simulink model "exam_model_R2020a_final"  (R2022a)
settings: Solver=VariableStepAuto  StartTime=0.0  StopTime=120  FixedStep=inc  MaxStep=1e-2  EnableMultiTasking=on
undefined symbols (not defined in the file): B, C, converter_const, J, ki, kiw, kp, kpw, kpw_load, L, L_f, R_f, R_L, T_load, Vin
settings Model: Creator=Dave  LastModifiedBy=aasav
settings SolverCC: AlgebraicLoopSolver=TrustRegion
settings DataIOCC: LimitDataPoints=on  SaveFormat=Array  SignalLoggingSaveFormat=ModelDataLogs  LoggingToFile=on
settings OptimizationCC: ExpressionDepthLimit=2147483647  InitFltsAndDblsToZero=on  LifeSpan=inf
settings DebuggingCC: SaveWithParameterizedLinksMsg=none  UnderspecifiedInitializationDetection=Classic  MergeDetectMultiDrivingBlocksExec=none  SolverPrmCheckMsg=warning  FcnCallInpInsideContextMsg=warning  UnconnectedInputMsg=warning  UnconnectedOutputMsg=warning  UnconnectedLineMsg=warning  StateNameClashWarn=warning  SFUnexpectedBacktrackingDiag=warning  SFNoUnconditionalDefaultTransitionDiag=warning  SFExecutionAtInitializationDiag=none  SFMachineParentedDataDiag=warning  ArithmeticOperatorsInVariantConditions=warning
settings HardwareCC: ProdBitPerPointer=32  ProdBitPerSizeT=32  ProdBitPerPtrDiffT=32  ProdLargestAtomicFloat=None  ProdIntDivRoundTo=Undefined  ProdEndianess=Unspecified  ProdWordSize=32  ProdHWDeviceType=32-bit Generic
settings ModelReferenceCC: PropagateSignalLabelsOutOfModel=off
settings CodeAppCC: StateflowObjectComments=on
settings GRTTargetCC: TargetLangStandard=C89/C90 (ANSI)  CombineOutputUpdateFcns=off  GRTInterface=on
settings ConfigComp: CovMetricSettings=dw  CovSaveCumulativeToWorkspaceVar=on  CovSaveSingleToWorkspaceVar=on

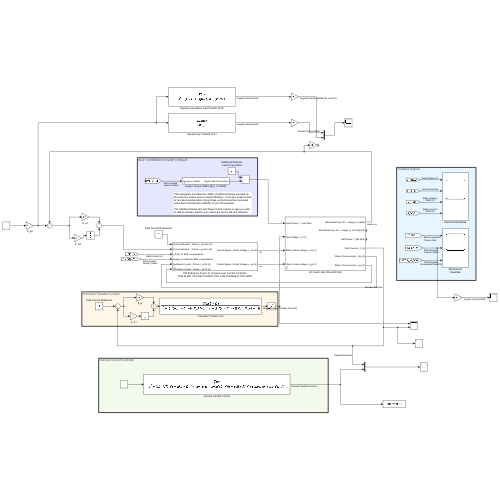
[thumbnail: Simulink's stored preview of the top-level diagram]
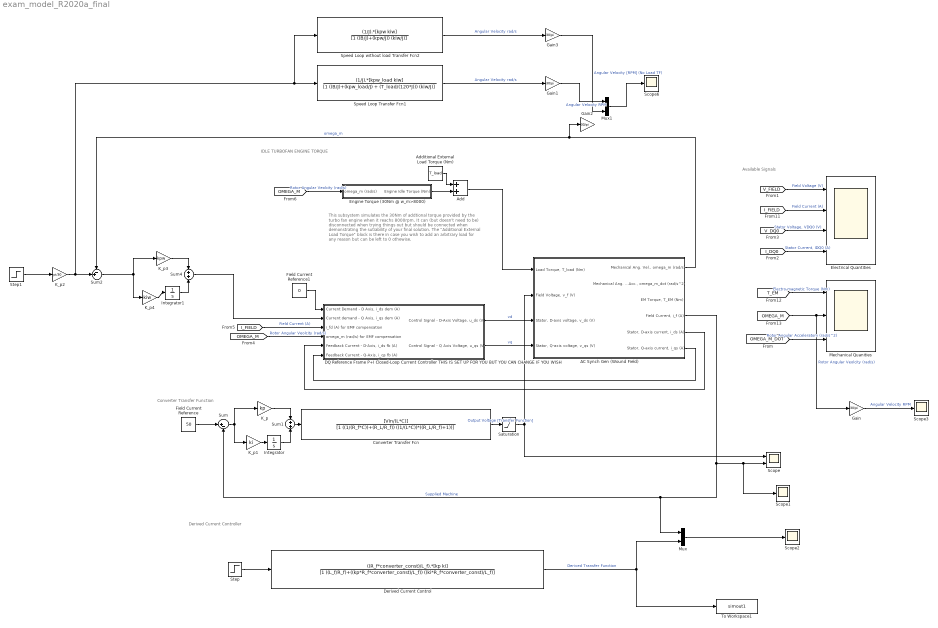
== system exam_model_R2020a_final ==
  note: Converter Transfer Function
  note: Derived Current Controller
  note: This subsystem simulates the 30Nm of addtional torque provided by the turbo fan engine when it reachs 8000rpm.  It can (but doesn't need to be) disconnected when trying things out but should be connected when demonstrating the sutiability of your final solution.
      |
      | The "Additional External Load Torque" block is there in case you wish to add an arbitrary load for any reason but can be left to 0 othewise.
  note: IDLE TURBOFAN ENGINE TORQUE
  note: Available Signals
  AC Synch Gen (Wound Field) : Subsystem  mask(Synchronous Generator Model (No Saturation)){J_rotor=0.5, B_viscous=0.05, Pole_Pairs=3, Ns_by_Nf=0.3, wind_const=1.5, R_s=0.04, L_s=5e-5, L_d=0.00057, R_fd_p=0.223*1.5*0.3^2, L_fd_p=0.0138*1.5*0.3^2, L_q=0.00032}
      mask prompts: J_rotor "Rotor Mass Moment-of-Interia, J_rotor, kg m^2"; B_viscous "Rotor Viscous Friction Coefficient, B_viscous (Nm s/rad)"; Pole_Pairs "Rotor Pole Pairs"; Ns_by_Nf "Stator to Field Turns Ratio, Ns_by_Nf"; wind_const "Winding Constant (Normally 1.5)"; R_s "Stator Resistance, R_s (Ohms)"; L_s "Stator Leakage Inductance, L_s (H)"; L_d "D-Axis Synchronous Inductance, L_d (H)"; R_fd_p "Referred Field Resistance, R_fd_p (Ohms)"; L_fd_p "Referred Field Leakage Inducatnce, L_fd_p (H)"; L_q "Q-Axis Synchronous Inductance, L_q (H)"
      mask help: Standard SI units version of a Would Field Synchronous Generator. All rotor parameters must be supplied referred from the rotor side to the stator.
      mask init:
      | L_md = L_d - L_s
      | L_MD_TOTAL = 1 / ( ( 1/L_md ) + ( 1/L_fd_p ) + ( 1/L_s ) )
      | L_mq = L_q - L_s
      | L_MQ_TOTAL = 1 / ( ( 1/L_mq ) + ( 1/L_s ) )
      mask DialogControl Container4 Prompt: Mechanical Parameters
      mask DialogControl Container6 Prompt: Electrical Parameters
      mask DialogControl Container8 Prompt: General
      mask DialogControl Container13 Prompt: Stator Synchronous Parameters
      mask DialogControl Container9 Prompt: D-Axis Parameters
      mask DialogControl Container11 Prompt: Referred Field Winding
      mask DialogControl Container10 Prompt: Q-Axis Parameters
  Add : Sum
  Additional External Load Torque (Nm) : Constant  Value=T_load
  Converter Transfer Fcn : TransferFcn  Numerator=[Vin/(L*C)]  Denominator=[1 ((1/(R_f*C))+(R_L/R_f)) ((1/(L*C))*((R_L/R_f)+1))]
  DQ Reference Frame P+I Closed-Loop Current Controller THIS IS SET UP FOR YOU BUT YOU CAN CHANGE IF YOU WISH : Subsystem  mask{emfcomp=on, kp_d=5, ki_d=20, kp_q=3, ki_q=15}
      mask prompts: emfcomp "Current Controller EMF Compensation?"; kp_d "d-Axis Proportional Gain"; ki_d "d-Axis Integral Gain"; kp_q "q-Axis Proportional Gain"; ki_q "q-axis Integral Gain"
      mask help:
      | A simple two axis feedback controller based upon a P + I structure.
      |
      | NOTE: The block simply implements two independent P + I controllers with no saturation or integrator anti-wind up protection.  Controller Gains are set in this dialog box.
      |
      | There is the option of using EMF Compesnation to simplfy controller design.  When enabled the EMF is added to the relevant axis of the machine winding to ensure that the controller is only providivng a voltage over and above this value, this simplifies controller design over a wide speed range.
      mask DialogControl Container5 Prompt: Current Controller
      mask DialogControl ParameterGroupVar Prompt: Current Controller Gains
      mask DialogControl Container4 Prompt: D-Axis P+I Controller Gains
      mask DialogControl Container3 Prompt: Q-Axis P+I Controller Gains
  Derived Current Control : TransferFcn  Numerator=((R_f*converter_const)/L_f).*[kp ki]  Denominator=[1 ((L_f/R_f)+((kp*R_f*converter_const)/L_f)) ((ki*R_f*converter_const)/L_f)]
  Electrical Quantities : Scope  NumInputPorts=4
  Engine Torque (30Nm @ w_m>8000) : Subsystem  mask(Engine Idle Torque Simulation (Once lit)){idle_speed=8000, idle_torque=30}
      mask prompts: idle_speed "Engine Ignition Speed (rev/min)"; idle_torque "Engine Idle Torque (Nm)"
      mask help:
      | This subsystem simulates the 30Nm of addtional torque provided by the turbo fan engine when the engine shaft reaches  8000rpm and the engine ignites.  It can (but doesn't need to be) disconnected when trying things out but should be connected when demonstrating the sutiability of your final solution.
      |
      | The "Additional External Load Torque" block is there in case you wish to add an arbitrary load for any reason but can be left to 0 othewise.
  Field Current Reference : Constant  Value=50
  Field Current Reference1 : Constant  Value=0
  Gain{,1..3} (4 alike) : Gain  Gain=30/pi
  Integrator : Integrator
  Integrator1 : Integrator
  K_p : Gain  Gain=kp
  K_p1 : Gain  Gain=ki
  K_p2 : Gain  Gain=pi/30
  K_p3 : Gain  Gain=kpw
  K_p4 : Gain  Gain=kiw
  Mechanical Quanities : Scope  NumInputPorts=3
  Mux : Mux  Inputs=2
  Mux1 : Mux  Inputs=2
  Saturation : Saturate  UpperLimit=Vin*0.9  LowerLimit=0
  Scope : Scope  NumInputPorts=2
  Scope{1..3,6} (4 alike) : Scope
  Speed Loop Transfer Fcn1 : TransferFcn  Numerator=(1/J).*[kpw_load kiw]  Denominator=[1 ((B/J)+(kpw_load/J) + (T_load/(120*J))) (kiw/J)]
  Speed Loop without load Transfer Fcn2 : TransferFcn  Numerator=(1/J).*[kpw kiw]  Denominator=[1 ((B/J)+(kpw/J)) (kiw/J)]
  Step : Step  Time=0  After=50  SampleTime=0
  Step1 : Step  Time=5  After=12000  SampleTime=0
  Sum : Sum  Inputs=|+-
  Sum1 : Sum  Inputs=+|+
  Sum2 : Sum  Inputs=-+|
  Sum4 : Sum  Inputs=+|+
  To Workspace1 : ToWorkspace  VariableName=simout1  SaveFormat=Timeseries  SampleTime=-1
  wires:
  [OMEGA_M_DOT] -> Mechanical Quanities/3  "Rotor Angular Acceleratom (rad/s^2)"
  [I_DQ0] -> Electrical Quantities/4  "Stator Current, IDQ0 (A)"
  [V_DQ0] -> Electrical Quantities/3  "Stator Voltage, VDQ0 (V)"
  [I_FIELD] -> Electrical Quantities/2  "Field Current (A)"
  [V_FIELD] -> Electrical Quantities/1  "Field Voltage (V)"
  [T_EM] -> Mechanical Quanities/1  "Electro-magnetic Torque (Nm)"
  [OMEGA_M] -> Gain/1, Mechanical Quanities/2  "Rotor Angular Veolcity (rad/s)"
  AC Synch Gen (Wound Field)/6("Stator, Q-axis current, i_qs (A)") -> DQ Reference Frame P+I Closed-Loop Current Controller THIS IS SET UP FOR YOU BUT YOU CAN CHANGE IF YOU WISH/6("Feedback Current - Q-Axis, i_qs fb (A)")
  AC Synch Gen (Wound Field)/5("Stator, D-axis current, i_ds (A)") -> DQ Reference Frame P+I Closed-Loop Current Controller THIS IS SET UP FOR YOU BUT YOU CAN CHANGE IF YOU WISH/5("Feedback Current - D-Axis, i_ds fb (A)")
  DQ Reference Frame P+I Closed-Loop Current Controller THIS IS SET UP FOR YOU BUT YOU CAN CHANGE IF YOU WISH/1("Control Signal - D-Axis Voltage, u_ds (V)") -> AC Synch Gen (Wound Field)/3("Stator, D-axis voltage, v_ds (V)")  "vd"
  DQ Reference Frame P+I Closed-Loop Current Controller THIS IS SET UP FOR YOU BUT YOU CAN CHANGE IF YOU WISH/2("Control Signal - Q Axis Voltage, u_qs (V)") -> AC Synch Gen (Wound Field)/4("Stator, Q-axis voltage, v_qs (V)")  "vq"
  Add/1 -> AC Synch Gen (Wound Field)/1("Load Torque, T_load (Nm)")
  Additional External Load Torque (Nm)/1 -> Add/1
  Engine Torque (30Nm @ w_m>8000)/1(Engine Idle Torque (Nm)) -> Add/2
  [OMEGA_M] -> DQ Reference Frame P+I Closed-Loop Current Controller THIS IS SET UP FOR YOU BUT YOU CAN CHANGE IF YOU WISH/4(omega_m (rad/s) for EMF compensation)  "Rotor Angular Veolcity (rad/s)"
  [I_FIELD] -> DQ Reference Frame P+I Closed-Loop Current Controller THIS IS SET UP FOR YOU BUT YOU CAN CHANGE IF YOU WISH/3(i_fd (A) for EMF compensation)  "Field Current (A)"
  [OMEGA_M] -> Engine Torque (30Nm @ w_m>8000)/1(omega_m (rad/s))  "Rotor Angular Veolcity (rad/s)"
  Converter Transfer Fcn/1 -> Saturation/1  "Output Voltage [Transfer Function]"
  AC Synch Gen (Wound Field)/4("Field Current, i_f (A)") -> Mux/1, Sum/2, Scope1/1, Scope/2  "Supplied Machine"
  Field Current Reference/1 -> Sum/1
  K_p/1 -> Sum1/1
  Sum1/1 -> Converter Transfer Fcn/1
  Saturation/1 -> AC Synch Gen (Wound Field)/2("Field Voltage, v_f (V)"), Scope/1
  Sum/1 -> K_p1/1, K_p/1
  Integrator/1 -> Sum1/2
  K_p1/1 -> Integrator/1
  Step/1 -> Derived Current Control/1
  Derived Current Control/1 -> Mux/2, To Workspace1/1  "Derived Transfer Function"
  Mux/1 -> Scope2/1
  K_p2/1 -> Speed Loop without load Transfer Fcn2/1, Speed Loop Transfer Fcn1/1, Sum2/2
  Step1/1 -> K_p2/1
  AC Synch Gen (Wound Field)/1("Mechanical Ang. Vel., omega_m (rad/s)") -> Gain2/1, Sum2/1  "omega_m"
  K_p3/1 -> Sum4/1
  Sum2/1 -> K_p4/1, K_p3/1
  Integrator1/1 -> Sum4/2
  K_p4/1 -> Integrator1/1
  Sum4/1 -> DQ Reference Frame P+I Closed-Loop Current Controller THIS IS SET UP FOR YOU BUT YOU CAN CHANGE IF YOU WISH/2("Current demand - Q Axis, i_qs dem (A)")
  Field Current Reference1/1 -> DQ Reference Frame P+I Closed-Loop Current Controller THIS IS SET UP FOR YOU BUT YOU CAN CHANGE IF YOU WISH/1("Current Demand - D Axis, i_ds dem (A)")
  Gain/1 -> Scope3/1  "Angular Velocity RPM"
  Speed Loop Transfer Fcn1/1 -> Gain1/1  "Angular Velocity rad/s"
  Gain1/1 -> Mux1/1  "Angular Velocity RPM"
  Mux1/1 -> Scope6/1
  Speed Loop without load Transfer Fcn2/1 -> Gain3/1  "Angular Velocity rad/s"
  Gain3/1 -> Mux1/2  "Angular Velocity [RPM] (No Load TF)"

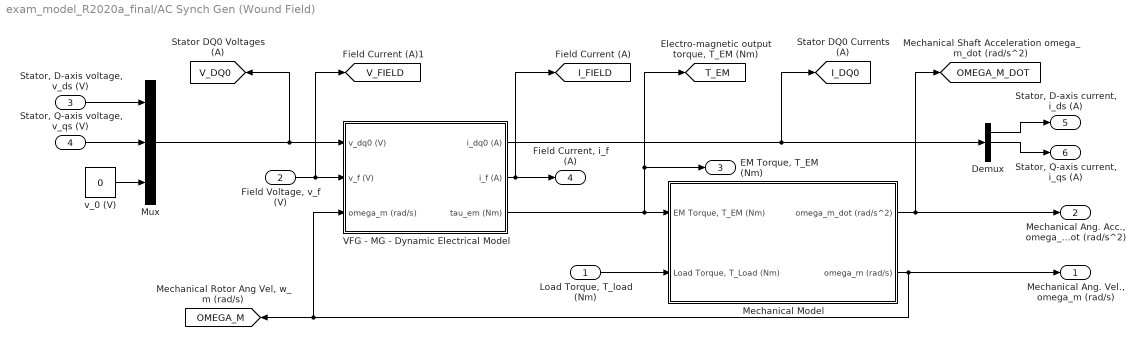
== system exam_model_R2020a_final/AC Synch Gen (Wound Field) ==
  "Load Torque, T_load (Nm)" : Inport
  "Field Voltage, v_f (V)" : Inport  Port=2
  "Stator, D-axis voltage, v_ds (V)" : Inport  Port=3
  "Stator, Q-axis voltage, v_qs (V)" : Inport  Port=4
  Demux : Demux  Outputs=3
  Mechanical Model : Subsystem  mask{Pole_Pairs=Pole_Pairs, J_rotor=J_rotor, B_viscous=B_viscous}
      mask prompts: Pole_Pairs "Rotor Pole Pairs"; J_rotor "Rotor Mass Moment-of-Inertia, J (kg m^2)"; B_viscous "Rotor Viscous Friction Constant, B_viscous (Nm s/rad)"
      mask DialogControl Container3 Prompt: Synchronous Generator Rotor Mechanical Parameters
  Mux : Mux  Inputs=3
  VFG - MG - Dynamic Electrical Model : Subsystem  mask{Pole_Pairs=Pole_Pairs, wind_const=wind_const, Ns_by_Nf=Ns_by_Nf, R_s=R_s, L_s=L_s, L_d=L_d, R_fd_p=R_fd_p, L_fd_p=L_fd_p, L_q=L_q}
      mask prompts: Pole_Pairs "Pole Pairs"; wind_const "Winding Constant"; Ns_by_Nf "Stator to Field Turns Ratio (Ns/Nf)"; R_s "Stator Resistance, R_s (Ohms)"; L_s "Stator Inductance, L_s (H)"; L_d "D-Axis Synchronous Inductance, L_d (H)"; R_fd_p "Referred Field Resistance, R_f_p (Ohms)"; L_fd_p "Referred Field Inductance, L_fd_p (H)"; L_q "Q-Axis Sychronous Inductance, L_q (H)"
      mask DialogControl Container4 Prompt: General Parameters
      mask DialogControl Container5 Prompt: D-Axis Parameters
      mask DialogControl Container8 Prompt: Referred Field
      mask DialogControl Container6 Prompt: Q-Axis Parameters
  v_0 (V) : Constant  Value=0
  "Mechanical Ang. Vel., omega_m (rad/s)" : Outport
  "Mechanical Ang. Acc., omega_m_dot (rad/s^2)" : Outport  Port=2
  "EM Torque, T_EM (Nm)" : Outport  Port=3
  "Field Current, i_f (A)" : Outport  Port=4
  "Stator, D-axis current, i_ds (A)" : Outport  Port=5
  "Stator, Q-axis current, i_qs (A)" : Outport  Port=6
  tag scope: I_DQ0=global, I_FIELD=global, OMEGA_M=global, OMEGA_M_DOT=global, T_EM=global, V_DQ0=global, V_FIELD=global
  wires:
  VFG - MG - Dynamic Electrical Model/1(i_dq0 (A)) -> Demux/1, [I_DQ0]
  "Field Voltage, v_f (V)"/1 -> [V_FIELD], VFG - MG - Dynamic Electrical Model/2(v_f (V))
  Mechanical Model/2(omega_m (rad/s)) -> [OMEGA_M], VFG - MG - Dynamic Electrical Model/3(omega_m (rad/s)), "Mechanical Ang. Vel., omega_m (rad/s)"/1
  VFG - MG - Dynamic Electrical Model/2(i_f (A)) -> [I_FIELD], "Field Current, i_f (A)"/1
  VFG - MG - Dynamic Electrical Model/3(tau_em (Nm)) -> [T_EM], "EM Torque, T_EM (Nm)"/1, Mechanical Model/1("EM Torque, T_EM (Nm)")
  "Load Torque, T_load (Nm)"/1 -> Mechanical Model/2("Load Torque, T_Load (Nm)")
  "Stator, D-axis voltage, v_ds (V)"/1 -> Mux/1
  "Stator, Q-axis voltage, v_qs (V)"/1 -> Mux/2
  v_0 (V)/1 -> Mux/3
  Mux/1 -> [V_DQ0], VFG - MG - Dynamic Electrical Model/1(v_dq0 (V))
  Demux/1 -> "Stator, D-axis current, i_ds (A)"/1
  Demux/2 -> "Stator, Q-axis current, i_qs (A)"/1
  Mechanical Model/1(omega_m_dot (rad/s^2)) -> [OMEGA_M_DOT], "Mechanical Ang. Acc., omega_m_dot (rad/s^2)"/1

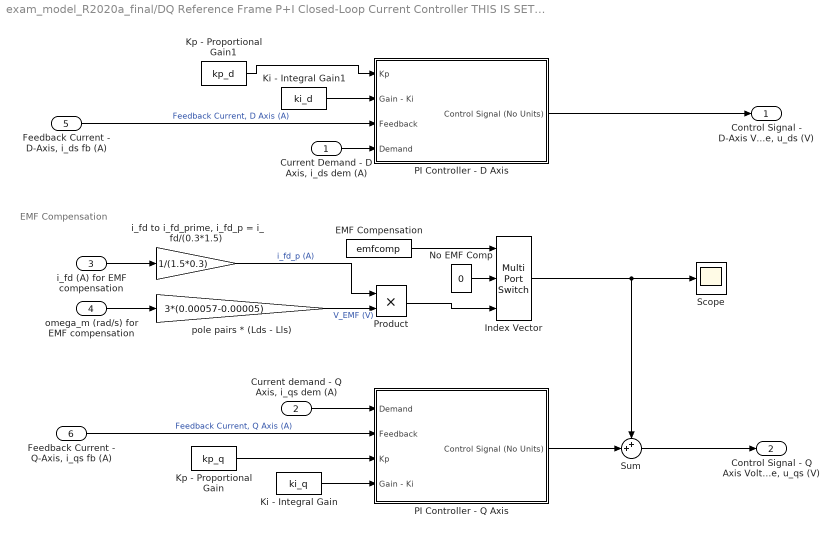
== system exam_model_R2020a_final/DQ Reference Frame P+I Closed-Loop Current Controller THIS IS SET UP FOR YOU BUT YOU CAN CHANGE IF YOU WISH ==
  note: EMF Compensation
  "Current Demand - D Axis, i_ds dem (A)" : Inport
  "Current demand - Q Axis, i_qs dem (A)" : Inport  Port=2
  i_fd (A) for EMF compensation : Inport  Port=3
  omega_m (rad/s) for EMF compensation : Inport  Port=4
  "Feedback Current - D-Axis, i_ds fb (A)" : Inport  Port=5
  "Feedback Current - Q-Axis, i_qs fb (A)" : Inport  Port=6
  EMF Compensation : Constant  Value=emfcomp
  Index Vector : MultiPortSwitch  DataPortOrder=Zero-based contiguous  Inputs=2  zeroidx=on  SaturateOnIntegerOverflow=off  InputSameDT=off
  Ki - Integral Gain : Constant  Value=ki_q
  Ki - Integral Gain1 : Constant  Value=ki_d
  Kp - Proportional Gain : Constant  Value=kp_q
  Kp - Proportional Gain1 : Constant  Value=kp_d
  No EMF Comp : Constant  Value=0
  PI Controller - D Axis : Subsystem  TreatAsAtomicUnit=on
  PI Controller - Q Axis : Subsystem  TreatAsAtomicUnit=on
  Product : Product
  Scope : Scope
  Sum : Sum  Inputs=++|
  "i_fd to i_fd_prime, i_fd_p = i_fd/(0.3*1.5)" : Gain  Gain=1/(1.5*0.3)
  pole pairs * (Lds - Lls) : Gain  Gain=3*(0.00057-0.00005)
  "Control Signal - D-Axis Voltage, u_ds (V)" : Outport  VectorParamsAs1DForOutWhenUnconnected=off
  "Control Signal - Q Axis Voltage, u_qs (V)" : Outport  Port=2  VectorParamsAs1DForOutWhenUnconnected=off
  wires:
  "Current demand - Q Axis, i_qs dem (A)"/1 -> PI Controller - Q Axis/1(Demand)
  "Feedback Current - Q-Axis, i_qs fb (A)"/1 -> PI Controller - Q Axis/2(Feedback)  "Feedback Current, Q Axis (A)"
  "Feedback Current - D-Axis, i_ds fb (A)"/1 -> PI Controller - D Axis/3(Feedback)  "Feedback Current, D Axis (A)"
  "Current Demand - D Axis, i_ds dem (A)"/1 -> PI Controller - D Axis/4(Demand)
  PI Controller - Q Axis/1(Control Signal (No Units)) -> Sum/2
  pole pairs * (Lds - Lls)/1 -> Product/2  "V_EMF (V)"
  Sum/1 -> "Control Signal - Q Axis Voltage, u_qs (V)"/1
  omega_m (rad/s) for EMF compensation/1 -> pole pairs * (Lds - Lls)/1
  EMF Compensation/1 -> Index Vector/1
  No EMF Comp/1 -> Index Vector/2
  Index Vector/1 -> Sum/1, Scope/1
  PI Controller - D Axis/1(Control Signal (No Units)) -> "Control Signal - D-Axis Voltage, u_ds (V)"/1
  Kp - Proportional Gain/1 -> PI Controller - Q Axis/3(Kp)
  Ki - Integral Gain/1 -> PI Controller - Q Axis/4(Gain - Ki)
  Kp - Proportional Gain1/1 -> PI Controller - D Axis/1(Kp)
  Ki - Integral Gain1/1 -> PI Controller - D Axis/2(Gain - Ki)
  i_fd (A) for EMF compensation/1 -> "i_fd to i_fd_prime, i_fd_p = i_fd/(0.3*1.5)"/1
  "i_fd to i_fd_prime, i_fd_p = i_fd/(0.3*1.5)"/1 -> Product/1  "i_fd_p (A)"
  Product/1 -> Index Vector/3

== system exam_model_R2020a_final/Engine Torque (30Nm @ w_m>8000) ==
  omega_m (rad/s) : Inport
  Engine Idle Torque Magnitude (Nm) : Constant  Value=idle_torque
  Engine Ignition Speed (rev/min) : Constant  Value=idle_speed
  Gain : Gain  Gain=2*pi/60
  Gain1 : Gain  Gain=-1
  Product : Product
  Relational Operator : RelationalOperator  OutDataTypeStr=boolean  RndMeth=Simplest  InputSameDT=off
  Engine Idle Torque (Nm) : Outport
  wires:
  Gain/1 -> Relational Operator/2
  Engine Idle Torque Magnitude (Nm)/1 -> Gain1/1
  Product/1 -> Engine Idle Torque (Nm)/1
  Relational Operator/1 -> Product/2
  omega_m (rad/s)/1 -> Relational Operator/1
  Engine Ignition Speed (rev/min)/1 -> Gain/1
  Gain1/1 -> Product/1

== system exam_model_R2020a_final/AC Synch Gen (Wound Field)/Mechanical Model ==
  note: T_Net = T_EM - T_Load
      | T_Net = (J * omega_m_dot) + (B * omega_m)
  "EM Torque, T_EM (Nm)" : Inport
  "Load Torque, T_Load (Nm)" : Inport  Port=2
  Gain : Gain  Gain=1/J_rotor
  Gain1 : Gain  Gain=B_viscous
  Integrator : Integrator
  Sum : Sum  Inputs=+--
  omega_m_dot (rad/s^2) : Outport
  omega_m (rad/s) : Outport  Port=2
  wires:
  "Load Torque, T_Load (Nm)"/1 -> Sum/2
  Sum/1 -> Gain/1  "Net Torque, T_net (Nm)"
  "EM Torque, T_EM (Nm)"/1 -> Sum/1
  Integrator/1 -> Gain1/1, omega_m (rad/s)/1  "omega_m (rad/s)"
  Gain/1 -> omega_m_dot (rad/s^2)/1, Integrator/1  "omega_m_dot (rad/s)"
  Gain1/1 -> Sum/3  "Viscous Friction Torque, T_fric (Nm)"

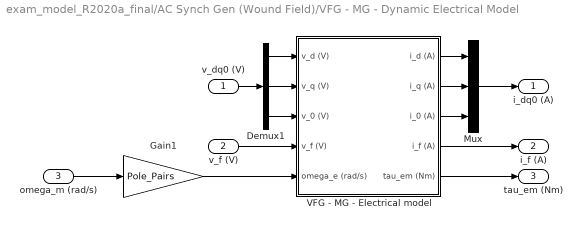
== system exam_model_R2020a_final/AC Synch Gen (Wound Field)/VFG - MG - Dynamic Electrical Model ==
  v_dq0 (V) : Inport
  v_f (V) : Inport  Port=2
  omega_m (rad/s) : Inport  Port=3
  Demux1 : Demux  Outputs=3
  Gain1 : Gain  Gain=Pole_Pairs
  Mux : Mux  Inputs=3
  VFG - MG - Electrical model : Subsystem
  i_dq0 (A) : Outport
  i_f (A) : Outport  Port=2
  tau_em (Nm) : Outport  Port=3
  wires:
  VFG - MG - Electrical model/4(i_f (A)) -> i_f (A)/1
  VFG - MG - Electrical model/5(tau_em (Nm)) -> tau_em (Nm)/1
  v_dq0 (V)/1 -> Demux1/1
  Mux/1 -> i_dq0 (A)/1
  omega_m (rad/s)/1 -> Gain1/1
  Gain1/1 -> VFG - MG - Electrical model/5(omega_e (rad/s))
  Demux1/1 -> VFG - MG - Electrical model/1(v_d (V))
  Demux1/2 -> VFG - MG - Electrical model/2(v_q (V))
  Demux1/3 -> VFG - MG - Electrical model/3(v_0 (V))
  v_f (V)/1 -> VFG - MG - Electrical model/4(v_f (V))
  VFG - MG - Electrical model/1(i_d (A)) -> Mux/1
  VFG - MG - Electrical model/2(i_q (A)) -> Mux/2
  VFG - MG - Electrical model/3(i_0 (A)) -> Mux/3

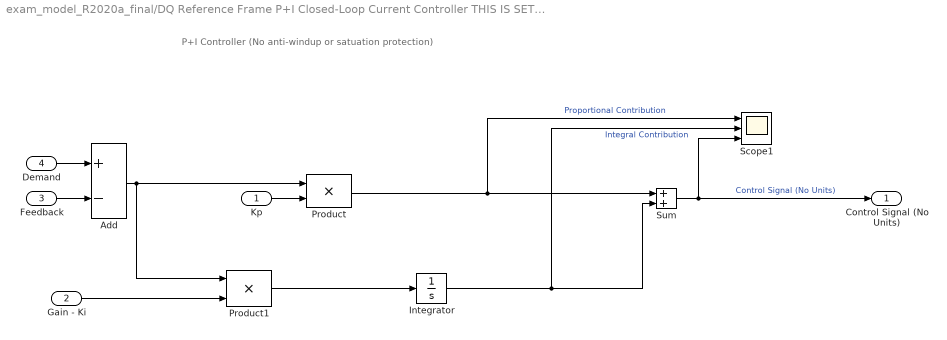
== system exam_model_R2020a_final/DQ Reference Frame P+I Closed-Loop Current Controller THIS IS SET UP FOR YOU BUT YOU CAN CHANGE IF YOU WISH/PI Controller - D Axis ==
  note: P+I Controller (No anti-windup or satuation protection)
  Kp : Inport
  Gain - Ki : Inport  Port=2
  Feedback : Inport  Port=3
  Demand : Inport  Port=4
  Add : Sum  Inputs=+-
  Integrator : Integrator
  Product : Product  InputSameDT=on  SaturateOnIntegerOverflow=on  OutDataTypeStr=Inherit: Same as first input
  Product1 : Product  InputSameDT=on  SaturateOnIntegerOverflow=on  OutDataTypeStr=Inherit: Same as first input
  Scope1 : Scope  NumInputPorts=3
  Sum : Sum  InputSameDT=on  SaturateOnIntegerOverflow=on  OutDataTypeStr=Inherit: Same as first input
  Control Signal (No Units) : Outport  VectorParamsAs1DForOutWhenUnconnected=off
  wires:
  Product1/1 -> Integrator/1
  Product/1 -> Scope1/1, Sum/1  "Proportional Contribution"
  Sum/1 -> Scope1/3, Control Signal (No Units)/1  "Control Signal (No Units)"
  Gain - Ki/1 -> Product1/2
  Kp/1 -> Product/2
  Demand/1 -> Add/1
  Feedback/1 -> Add/2
  Add/1 -> Product1/1, Product/1
  Integrator/1 -> Scope1/2, Sum/2  "Integral Contribution"

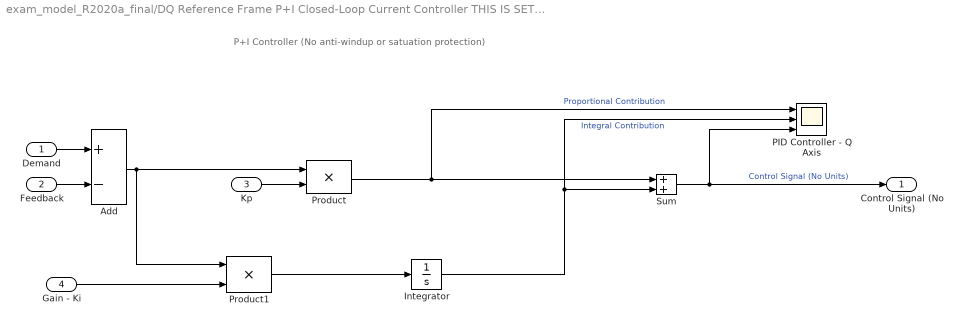
== system exam_model_R2020a_final/DQ Reference Frame P+I Closed-Loop Current Controller THIS IS SET UP FOR YOU BUT YOU CAN CHANGE IF YOU WISH/PI Controller - Q Axis ==
  note: P+I Controller (No anti-windup or satuation protection)
  Demand : Inport
  Feedback : Inport  Port=2
  Kp : Inport  Port=3
  Gain - Ki : Inport  Port=4
  Add : Sum  Inputs=+-
  Integrator : Integrator
  PID Controller - Q Axis : Scope  NumInputPorts=3
  Product : Product  InputSameDT=on  SaturateOnIntegerOverflow=on  OutDataTypeStr=Inherit: Same as first input
  Product1 : Product  InputSameDT=on  SaturateOnIntegerOverflow=on  OutDataTypeStr=Inherit: Same as first input
  Sum : Sum  InputSameDT=on  SaturateOnIntegerOverflow=on  OutDataTypeStr=Inherit: Same as first input
  Control Signal (No Units) : Outport  VectorParamsAs1DForOutWhenUnconnected=off
  wires:
  Add/1 -> Product1/1, Product/1
  Feedback/1 -> Add/2
  Demand/1 -> Add/1
  Kp/1 -> Product/2
  Gain - Ki/1 -> Product1/2
  Sum/1 -> PID Controller - Q Axis/3, Control Signal (No Units)/1  "Control Signal (No Units)"
  Product/1 -> PID Controller - Q Axis/1, Sum/1  "Proportional Contribution"
  Product1/1 -> Integrator/1
  Integrator/1 -> Sum/2, PID Controller - Q Axis/2  "Integral Contribution"

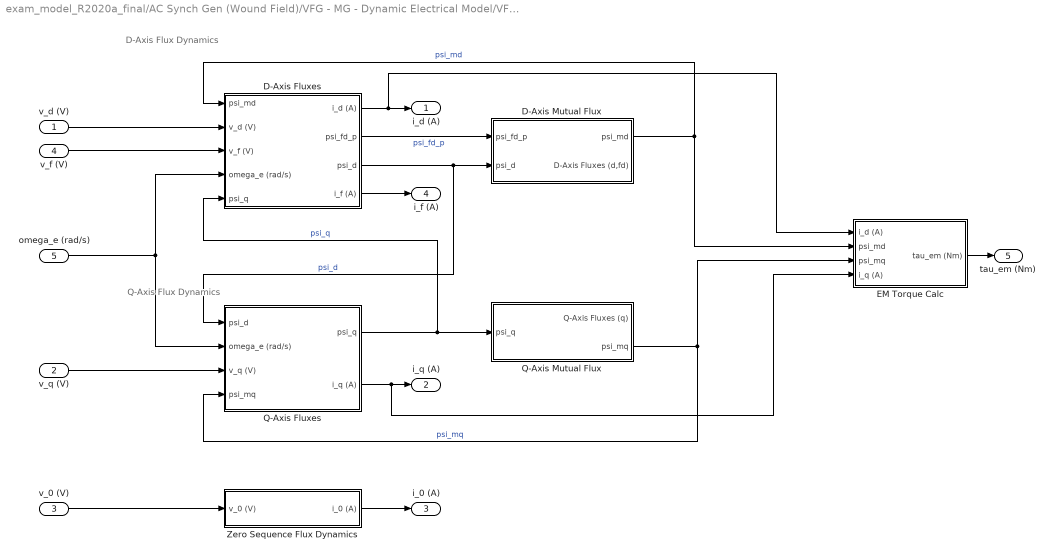
== system exam_model_R2020a_final/AC Synch Gen (Wound Field)/VFG - MG - Dynamic Electrical Model/VFG - MG - Electrical model ==
  note: Q-Axis Flux Dynamics
  note: D-Axis Flux Dynamics
  v_d (V) : Inport
  v_q (V) : Inport  Port=2
  v_0 (V) : Inport  Port=3
  v_f (V) : Inport  Port=4
  omega_e (rad/s) : Inport  Port=5
  D-Axis Fluxes : Subsystem
  D-Axis Mutual Flux : Subsystem
  EM Torque Calc : Subsystem
  Q-Axis Fluxes : Subsystem
  Q-Axis Mutual Flux : Subsystem
  Zero Sequence Flux Dynamics : Subsystem
  i_d (A) : Outport
  i_q (A) : Outport  Port=2
  i_0 (A) : Outport  Port=3
  i_f (A) : Outport  Port=4
  tau_em (Nm) : Outport  Port=5
  wires:
  v_d (V)/1 -> D-Axis Fluxes/2(v_d (V))
  Q-Axis Fluxes/1(psi_q) -> D-Axis Fluxes/5(psi_q), Q-Axis Mutual Flux/1(psi_q)  "psi_q"
  v_q (V)/1 -> Q-Axis Fluxes/3(v_q (V))
  omega_e (rad/s)/1 -> Q-Axis Fluxes/2(omega_e (rad/s)), D-Axis Fluxes/4(omega_e (rad/s))
  v_f (V)/1 -> D-Axis Fluxes/3(v_f (V))
  D-Axis Fluxes/4(i_f (A)) -> i_f (A)/1
  EM Torque Calc/1(tau_em (Nm)) -> tau_em (Nm)/1
  D-Axis Fluxes/3(psi_d) -> Q-Axis Fluxes/1(psi_d), D-Axis Mutual Flux/2(psi_d)  "psi_d"
  v_0 (V)/1 -> Zero Sequence Flux Dynamics/1(v_0 (V))
  Zero Sequence Flux Dynamics/1(i_0 (A)) -> i_0 (A)/1
  D-Axis Fluxes/2(psi_fd_p) -> D-Axis Mutual Flux/1(psi_fd_p)  "psi_fd_p"
  D-Axis Fluxes/1(i_d (A)) -> EM Torque Calc/1(i_d (A)), i_d (A)/1
  Q-Axis Mutual Flux/2(psi_mq) -> Q-Axis Fluxes/4(psi_mq), EM Torque Calc/3(psi_mq)  "psi_mq"
  Q-Axis Fluxes/2(i_q (A)) -> EM Torque Calc/4(i_q (A)), i_q (A)/1
  D-Axis Mutual Flux/1(psi_md) -> EM Torque Calc/2(psi_md), D-Axis Fluxes/1(psi_md)  "psi_md"

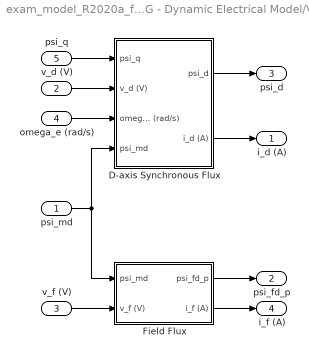
== system exam_model_R2020a_final/AC Synch Gen (Wound Field)/VFG - MG - Dynamic Electrical Model/VFG - MG - Electrical model/D-Axis Fluxes ==
  psi_md : Inport
  v_d (V) : Inport  Port=2
  v_f (V) : Inport  Port=3
  omega_e (rad/s) : Inport  Port=4
  psi_q : Inport  Port=5
  D-axis Synchronous Flux : Subsystem
  Field Flux : Subsystem
  i_d (A) : Outport
  psi_fd_p : Outport  Port=2
  psi_d : Outport  Port=3
  i_f (A) : Outport  Port=4
  wires:
  D-axis Synchronous Flux/1(psi_d) -> psi_d/1
  v_d (V)/1 -> D-axis Synchronous Flux/2(v_d (V))
  omega_e (rad/s)/1 -> D-axis Synchronous Flux/3(omega_e (rad/s))
  psi_md/1 -> Field Flux/1(psi_md), D-axis Synchronous Flux/4(psi_md)
  psi_q/1 -> D-axis Synchronous Flux/1(psi_q)
  Field Flux/1(psi_fd_p) -> psi_fd_p/1
  v_f (V)/1 -> Field Flux/2(v_f (V))
  Field Flux/2(i_f (A)) -> i_f (A)/1
  D-axis Synchronous Flux/2(i_d (A)) -> i_d (A)/1

== system exam_model_R2020a_final/AC Synch Gen (Wound Field)/VFG - MG - Dynamic Electrical Model/VFG - MG - Electrical model/D-Axis Mutual Flux ==
  note: psi_md = L_MD_TOTAL * (psi_d / L_s + psi_fd / L_fd_p)
  psi_fd_p : Inport
  psi_d : Inport  Port=2
  Gain : Gain  Gain=1/L_s
  Gain2 : Gain  Gain=1/L_fd_p
  Gain3 : Gain  Gain=L_MD_TOTAL
  Mux : Mux  Inputs=2
  Sum2 : Sum  Inputs=2
  psi_md : Outport
  D-Axis Fluxes (d,fd) : Outport  Port=2
  wires:
  Gain/1 -> Sum2/1
  Gain2/1 -> Sum2/2
  psi_d/1 -> Gain/1, Mux/1
  Sum2/1 -> Gain3/1
  Gain3/1 -> psi_md/1  "psi_md"
  Mux/1 -> D-Axis Fluxes (d,fd)/1
  psi_fd_p/1 -> Gain2/1, Mux/2

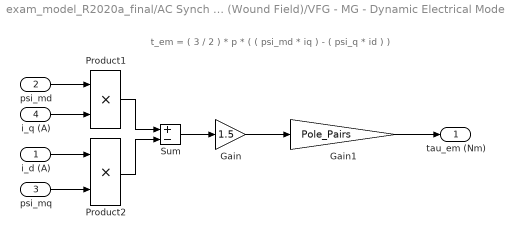
== system exam_model_R2020a_final/AC Synch Gen (Wound Field)/VFG - MG - Dynamic Electrical Model/VFG - MG - Electrical model/EM Torque Calc ==
  note: t_em = ( 3 / 2 ) * p * ( ( psi_md * iq ) - ( psi_q * id ) )
  i_d (A) : Inport
  psi_md : Inport  Port=2
  psi_mq : Inport  Port=3
  i_q (A) : Inport  Port=4
  Gain : Gain  Gain=1.5
  Gain1 : Gain  Gain=Pole_Pairs
  Product1 : Product  RndMeth=Zero
  Product2 : Product  RndMeth=Zero
  Sum : Sum  Inputs=+-
  tau_em (Nm) : Outport
  wires:
  Product1/1 -> Sum/1
  Product2/1 -> Sum/2
  Sum/1 -> Gain/1
  psi_md/1 -> Product1/1
  i_q (A)/1 -> Product1/2
  i_d (A)/1 -> Product2/1
  psi_mq/1 -> Product2/2
  Gain/1 -> Gain1/1
  Gain1/1 -> tau_em (Nm)/1

== system exam_model_R2020a_final/AC Synch Gen (Wound Field)/VFG - MG - Dynamic Electrical Model/VFG - MG - Electrical model/Q-Axis Fluxes ==
  psi_d : Inport
  omega_e (rad/s) : Inport  Port=2
  v_q (V) : Inport  Port=3
  psi_mq : Inport  Port=4
  Q-axis Synchronous Flux : Subsystem
  psi_q : Outport
  i_q (A) : Outport  Port=2
  wires:
  Q-axis Synchronous Flux/1(psi_q) -> psi_q/1
  v_q (V)/1 -> Q-axis Synchronous Flux/2(v_q (V))
  psi_d/1 -> Q-axis Synchronous Flux/3(psi_d)
  omega_e (rad/s)/1 -> Q-axis Synchronous Flux/1(omega_e (rad/s))
  Q-axis Synchronous Flux/2(i_q (A)) -> i_q (A)/1
  psi_mq/1 -> Q-axis Synchronous Flux/4(psi_mq)

== system exam_model_R2020a_final/AC Synch Gen (Wound Field)/VFG - MG - Dynamic Electrical Model/VFG - MG - Electrical model/Q-Axis Mutual Flux ==
  note: psi_mq = L_MQ_TOTAL * (psi_q / L_s )
  psi_q : Inport
  Gain1 : Gain  Gain=1/L_s
  Gain3 : Gain  Gain=L_MQ_TOTAL
  Q-Axis Fluxes (q) : Outport
  psi_mq : Outport  Port=2
  wires:
  Gain3/1 -> psi_mq/1  "psi_mq"
  Gain1/1 -> Gain3/1
  psi_q/1 -> Q-Axis Fluxes (q)/1, Gain1/1

== system exam_model_R2020a_final/AC Synch Gen (Wound Field)/VFG - MG - Dynamic Electrical Model/VFG - MG - Electrical model/Zero Sequence Flux Dynamics ==
  note: d_by_dt(psi_zero) = v_zero - (r_s/l_s) * psi_zero
  v_0 (V) : Inport
  Gain1 : Gain  Gain=R_s
  Gain2 : Gain  Gain=1/L_s
  Integrator : Integrator
  Sum : Sum  Inputs=+-
  i_0 (A) : Outport
  wires:
  Sum/1 -> Integrator/1  "d_by_dt (psi_0)"
  v_0 (V)/1 -> Sum/1
  Integrator/1 -> Gain2/1  "psi_0"
  Gain1/1 -> Sum/2
  Gain2/1 -> i_0 (A)/1, Gain1/1  "i_0 (A)"

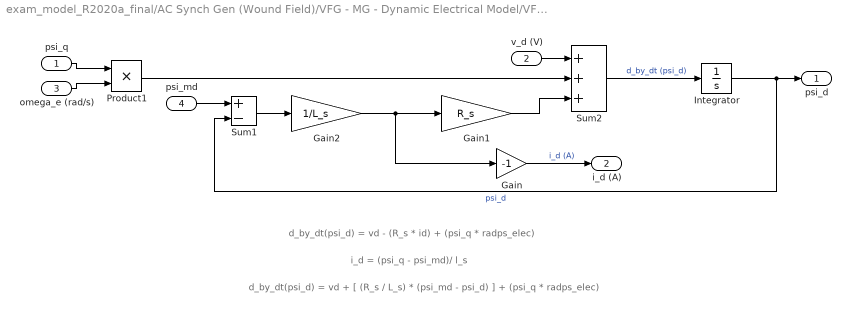
== system exam_model_R2020a_final/AC Synch Gen (Wound Field)/VFG - MG - Dynamic Electrical Model/VFG - MG - Electrical model/D-Axis Fluxes/D-axis Synchronous Flux ==
  note: d_by_dt(psi_d) = vd + [ (R_s / L_s) * (psi_md - psi_d) ] + (psi_q * radps_elec)
  note: d_by_dt(psi_d) = vd - (R_s * id) + (psi_q * radps_elec)
  note: i_d = (psi_q - psi_md)/ l_s
  psi_q : Inport
  v_d (V) : Inport  Port=2
  omega_e (rad/s) : Inport  Port=3
  psi_md : Inport  Port=4
  Gain : Gain  Gain=-1
  Gain1 : Gain  Gain=R_s
  Gain2 : Gain  Gain=1/L_s
  Integrator : Integrator
  Product1 : Product  RndMeth=Zero
  Sum1 : Sum  Inputs=+-
  Sum2 : Sum  Inputs=+++
  psi_d : Outport
  i_d (A) : Outport  Port=2
  wires:
  Sum1/1 -> Gain2/1
  Product1/1 -> Sum2/2
  Sum2/1 -> Integrator/1  "d_by_dt (psi_d)"
  v_d (V)/1 -> Sum2/1
  Integrator/1 -> psi_d/1, Sum1/2  "psi_d"
  psi_q/1 -> Product1/1
  omega_e (rad/s)/1 -> Product1/2
  psi_md/1 -> Sum1/1
  Gain1/1 -> Sum2/3
  Gain/1 -> i_d (A)/1  "i_d (A)"
  Gain2/1 -> Gain1/1, Gain/1

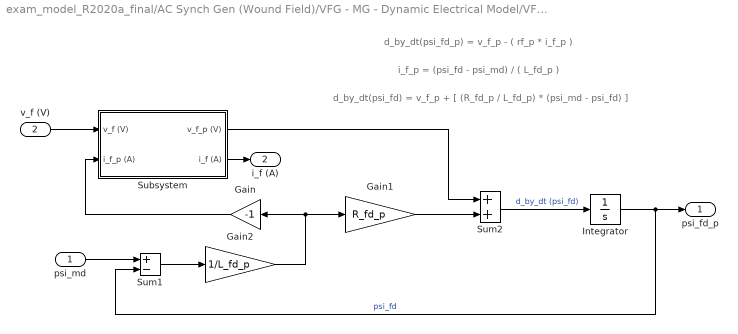
== system exam_model_R2020a_final/AC Synch Gen (Wound Field)/VFG - MG - Dynamic Electrical Model/VFG - MG - Electrical model/D-Axis Fluxes/Field Flux ==
  note: d_by_dt(psi_fd_p) = v_f_p - ( rf_p * i_f_p )
  note: i_f_p = (psi_fd - psi_md) / ( L_fd_p )
  note: d_by_dt(psi_fd) = v_f_p + [ (R_fd_p / L_fd_p) * (psi_md - psi_fd) ]
  psi_md : Inport
  v_f (V) : Inport  Port=2
  Gain : Gain  Gain=-1
  Gain1 : Gain  Gain=R_fd_p
  Gain2 : Gain  Gain=1/L_fd_p
  Integrator : Integrator
  Subsystem : Subsystem
  Sum1 : Sum  Inputs=+-
  Sum2 : Sum
  psi_fd_p : Outport
  i_f (A) : Outport  Port=2
  wires:
  Integrator/1 -> psi_fd_p/1, Sum1/2  "psi_fd"
  Gain1/1 -> Sum2/2
  Sum2/1 -> Integrator/1  "d_by_dt (psi_fd)"
  Subsystem/1(v_f_p (V)) -> Sum2/1
  psi_md/1 -> Sum1/1
  Sum1/1 -> Gain2/1
  Gain2/1 -> Gain1/1, Gain/1
  Gain/1 -> Subsystem/2(i_f_p (A))
  v_f (V)/1 -> Subsystem/1(v_f (V))
  Subsystem/2(i_f (A)) -> i_f (A)/1

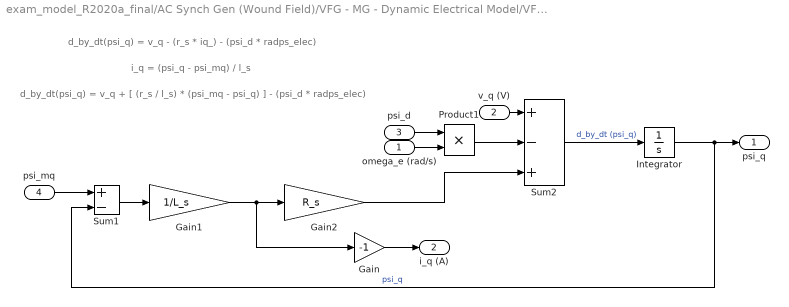
== system exam_model_R2020a_final/AC Synch Gen (Wound Field)/VFG - MG - Dynamic Electrical Model/VFG - MG - Electrical model/Q-Axis Fluxes/Q-axis Synchronous Flux ==
  note: d_by_dt(psi_q) = v_q + [ (r_s / l_s) * (psi_mq - psi_q) ] - (psi_d * radps_elec)
  note: d_by_dt(psi_q) = v_q - (r_s * iq_) - (psi_d * radps_elec)
  note: i_q = (psi_q - psi_mq) / l_s
  omega_e (rad/s) : Inport
  v_q (V) : Inport  Port=2
  psi_d : Inport  Port=3
  psi_mq : Inport  Port=4
  Gain : Gain  Gain=-1
  Gain1 : Gain  Gain=1/L_s
  Gain2 : Gain  Gain=R_s
  Integrator : Integrator
  Product1 : Product  RndMeth=Zero
  Sum1 : Sum  Inputs=+-
  Sum2 : Sum  Inputs=+-+
  psi_q : Outport
  i_q (A) : Outport  Port=2
  wires:
  omega_e (rad/s)/1 -> Product1/2
  psi_d/1 -> Product1/1
  Integrator/1 -> psi_q/1, Sum1/2  "psi_q"
  v_q (V)/1 -> Sum2/1
  Sum2/1 -> Integrator/1  "d_by_dt (psi_q)"
  Product1/1 -> Sum2/2
  Gain2/1 -> Sum2/3
  psi_mq/1 -> Sum1/1
  Sum1/1 -> Gain1/1
  Gain1/1 -> Gain2/1, Gain/1
  Gain/1 -> i_q (A)/1

== system exam_model_R2020a_final/AC Synch Gen (Wound Field)/VFG - MG - Dynamic Electrical Model/VFG - MG - Electrical model/D-Axis Fluxes/Field Flux/Subsystem ==
  note: i_f (A) = ( wind_const ) * (Ns_by_Nf) * i_f_p
  note: vfield_p = Ns_by_Nf * ( v(fieldp) - v(fieldn) )
  v_f (V) : Inport
  i_f_p (A) : Inport  Port=2
  Gain : Gain  Gain=wind_const
  Gain1 : Gain  Gain=Ns_by_Nf
  Gain2 : Gain  Gain=Ns_by_Nf
  v_f_p (V) : Outport
  i_f (A) : Outport  Port=2
  wires:
  v_f (V)/1 -> Gain1/1
  Gain2/1 -> i_f (A)/1
  Gain1/1 -> v_f_p (V)/1  "v_f_p (V)"
  i_f_p (A)/1 -> Gain/1
  Gain/1 -> Gain2/1
